simulink model "aurix_mbd_test"  (R2019a)
settings: Solver=FixedStepAuto  StartTime=0.0  StopTime=10.0  RelTol=1e-3
model workspace (MAT data in the model file):
  Ts = Simulink.Parameter
  Ts.Value = 0.005
  Ts.DataType = 'auto'
  Ts.Dimensions = [1 1]
libraries: sb275basic_lib x4, aurixappcontrollib x2
settings Model: Creator=seanryu  LastModifiedBy=seanryu
settings OptimizationCC: DefaultParameterBehavior=Inlined  EnhancedBackFolding=on  PassReuseOutputArgsAs=Individual arguments  OptimizeBlockOrder=speed  DifferentSizesBufferReuse=on  OptimizationCustomize=off
settings DebuggingCC: ParameterTunabilityLossMsg=error
settings HardwareCC: ProdBitPerPointer=32  ProdBitPerSizeT=32  ProdBitPerPtrDiffT=32  ProdLargestAtomicFloat=None  ProdWordSize=32  ProdHWDeviceType=Infineon->TriCore
settings SFSimCC: MATLABDynamicMemAlloc=off
settings RTWCC: SystemTargetFile=aurix_sys_trgt.tlc  TemplateMakefile=aurix_sys_trgt.tmf  Description=AURIX Target  GenerateReport=on  IncludeHyperlinkInReport=on  LaunchReport=on  GenerateTraceInfo=on  GenerateTraceReport=on  GenerateTraceReportSl=on  GenerateTraceReportSf=on  GenerateTraceReportEml=on
settings CodeAppCC: ForceParamTrailComments=on  IgnoreCustomStorageClasses=off  OperatorAnnotations=on  SimulinkDataObjDesc=on  SFDataObjDesc=on  InsertBlockDesc=on
settings STFCustomTargetCC: TargetLangStandard=C99 (ISO)  MultiwordLength=256  GenerateSampleERTMain=on  ModelReferenceCompliant=off  CombineOutputUpdateFcns=on  ERTCustomFileBanners=on  SupportContinuousTime=off  SupportNonInlinedSFcns=off  RemoveResetFunc=on  MATLABClassNameForMDSCustomization=Simulink.SoftwareTarget.ERTCustomization  GRTInterface=off  SystemTargetFile=aurix_sys_trgt.tlc
settings ERTTargetCC: TargetLangStandard=C99 (ISO)  GenerateSampleERTMain=on  ModelReferenceCompliant=off  ParMdlRefBuildCompliant=off  CompOptLevelCompliant=off  ConcurrentExecutionCompliant=off  ModelStepFunctionPrototypeControlCompliant=off  CPPClassGenCompliant=off  UseToolchainInfoCompliant=off  InlinedParameterPlacement=NonHierarchical  ERTCustomFileTemplate=aurix_sys_trgt_process.tlc

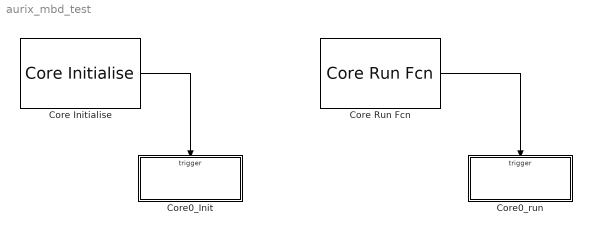
== system aurix_mbd_test ==
  Core Initialise : aurixappcontrollib/Core Initialise  pCore=0  pGlobInt=Pre Interrupt Enable  pUpdate=189
      settings: SourceProductName=Hitex AURIX Support Package
  Core Run Fcn : aurixappcontrollib/Core Run Fcn  pCore=0  pSchedule=0.01  pUpdate=205  pBlockPath=C:\00_Works\aurix_target
      settings: SourceProductName=Hitex AURIX Support Package
  Core0_Init : Subsystem  TreatAsAtomicUnit=on
  Core0_run : Subsystem  TreatAsAtomicUnit=on
  wires:
  Core Initialise/1 -> Core0_Init/Trigger
  Core Run Fcn/1 -> Core0_run/Trigger

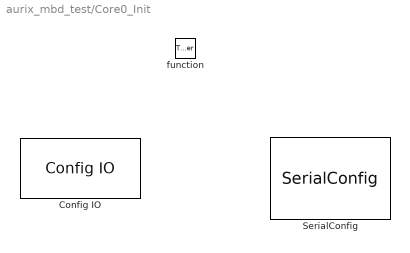
== system aurix_mbd_test/Core0_Init ==
  function : TriggerPort  TriggerType=function-call  VariantControl=Variant
  Config IO : sb275basic_lib/Config IO  pUpdate=4341  pPin0=GPIO Input  pPin1=GPIO Input  pPin2=GPIO Input  pPin3=GPIO Input  pPin4=GPIO Input  pPin5=GPIO Input  pPin6=GPIO Input  pPin7=GPIO Input  pPin8=GPIO Input  pPin9=GPIO Input  pPin10=GPIO Input  pPin11=GPIO Input  pPin12=GPIO Input  pPin13=GPIO Output  pPin14=GPIO Input  pPin15=GPIO Input  pPin16=GPIO Input  pPin17=GPIO Input  pPin18=GPIO Input  pPin19=GPIO Input  pPin20=GPIO Input  pPin21=GPIO Input  pPin22=GPIO Input  pPin23=GPIO Input  pPin24=GPIO Input  pPin25=GPIO Input  pPin26=GPIO Input  pPin27=GPIO Input  pPin28=GPIO Input  pPin29=GPIO Input  pPin30=GPIO Input  pPin31=GPIO Input  pPin32=GPIO Input  pPin33=GPIO Input  pPin34=GPIO Input  pPin35=GPIO Input  pPin36=GPIO Input  pPin37=GPIO Input  pPin38=GPIO Input  pPin39=GPIO Input  pPin40=GPIO Input  pPin41=GPIO Input  pPin42=GPIO Input  pPin43=GPIO Input  pPin44=GPIO Input  pPin45=GPIO Input  pPin46=GPIO Input  pPin47=GPIO Input  pPin48=GPIO Input  pPin49=GPIO Input  pPin50=GPIO Input  pPin51=GPIO Input
      settings: SourceProductName=Hitex AURIX Support Package
  SerialConfig : sb275basic_lib/SerialConfig  pBaud=115200  pUpdate=80
      settings: SourceProductName=Hitex AURIX Support Package

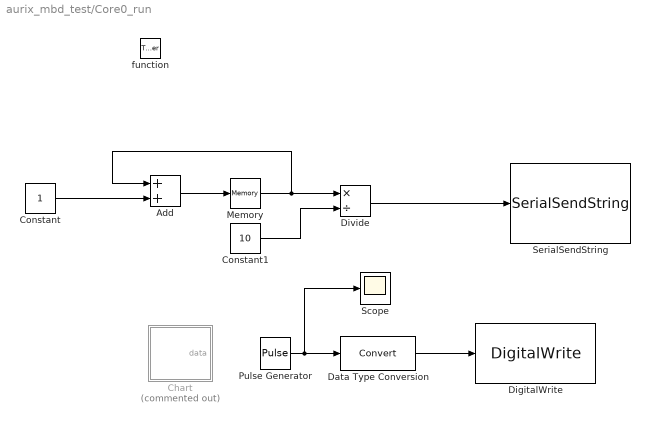
== system aurix_mbd_test/Core0_run ==
  function : TriggerPort  TriggerType=function-call  VariantControl=Variant  SampleTime=-1
  Add : Sum
  Chart : Stateflow chart  Commented=on  BlockKeywords=__PRM__SERIALIZED__DATA__:Stateflow Chart,Stateflow Diagram  TreatAsAtomicUnit=on
  Constant : Constant
  Constant1 : Constant  Value=10
  Data Type Conversion : DataTypeConversion
  DigitalWrite : sb275basic_lib/DigitalWrite  pNumber=13  pAction=From Model  pUpdate=133
      settings: SourceProductName=Hitex AURIX Support Package
  Divide : Product  Inputs=*/  OutDataTypeStr=Inherit: Inherit via back propagation
  Memory : Memory  InheritSampleTime=on
  Pulse Generator : DiscretePulseGenerator  Period=40  PulseWidth=20  SampleTime=-1
  Scope : Scope
  SerialSendString : sb275basic_lib/SerialSendString  pFmt=%2.2f\r\n  pUpdate=73
      settings: SourceProductName=Hitex AURIX Support Package
  wires:
  Constant/1 -> Add/2
  Add/1 -> Memory/1
  Memory/1 -> Add/1, Divide/1
  Constant1/1 -> Divide/2
  Divide/1 -> SerialSendString/1
  Pulse Generator/1 -> Scope/1, Data Type Conversion/1
  Data Type Conversion/1 -> DigitalWrite/1

== stateflow chart aurix_mbd_test/Core0_run/Chart ==
  state ON
    en:
    TimeCnt = 0;
    du:
    data = 1;
    TimeCnt = TimeCnt + 1;
  state OFF
    en:
    TimeCnt = 0;
    du:
    data = 0;
    TimeCnt = TimeCnt + 1;
  (default) -> ON
  OFF -> ON : [TimeCnt>99]
  ON -> OFF : [TimeCnt>99]
  data: data output; TimeCnt local
